simulink model "untitled1"  (R2022b)
settings: Solver=ode4  StartTime=0.0  StopTime=2  FixedStep=.01  RelTol=1e-3
settings Model: Creator=hp_desktop  LastModifiedBy=hp_desktop

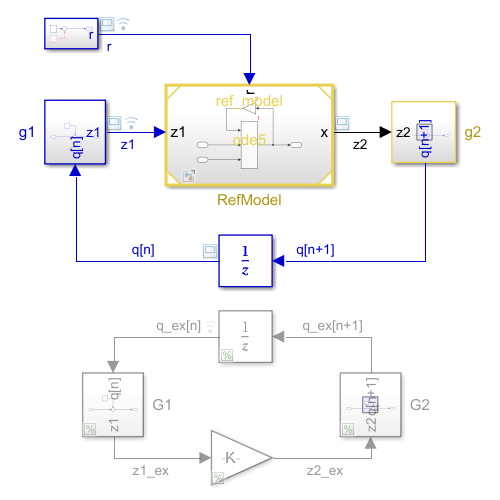
[thumbnail: Simulink's stored preview of the top-level diagram]
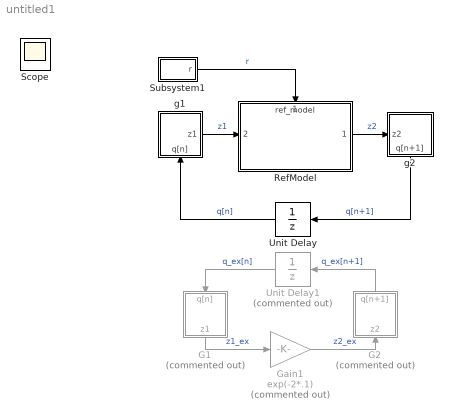
== system untitled1 ==
  G1 : Subsystem  Commented=on
      settings: PortSchema="{\"entries\":[{\"content\":{\"sides\":[{\"content\":{\"connectorIds\":[]},\"type\":\"ConnectorPlacement.EquallySpacedRectSide\",\"uuid\":\"86c8c839-e474-4a95-956c-b3cf1d577c6b\"},{\"content\":{\"connectorIds\":[],\"side\":\"RIGHT\"},\"type\":\"ConnectorPlacement.EquallySpacedRectSide\",\"uuid\":\"39481f83-4199-4de7-a4e8-5561103d4776\"},{\"content\":{\"connectorIds\":[\"Out1\"],\"side\":\"TOP\"},\"type\":\"ConnectorPlacement.EquallySpacedRectSide\",\"uuid\":\"ba4267bb-ac31-48a1-9c03-9fbc1cd5a7ee\"},{\"content\":{\"connectorIds\":[\"In1\"],\"side\":\"BOTTOM\"},\"type\":\"ConnectorPlacement.EquallySpacedRectSide\",\"uuid\":\"8bb6862b-83a9-47f6-8568-3761b0d351a6\"}]},\"type\":\"ConnectorPlacement.EquallySpacedConnector\",\"uuid\":\"7828d7b7-bf8b-4dbd-a99c-1d2acdedce65\"}],\"packageUris\":[\"http://schema.mathworks.com/mf0/Connector/R2020b\"],\"version\":\"1.0\"}"
  G2 : Subsystem  Commented=on
      settings: PortSchema="{\"entries\":[{\"content\":{\"sides\":[{\"content\":{\"connectorIds\":[]},\"type\":\"ConnectorPlacement.EquallySpacedRectSide\",\"uuid\":\"86c8c839-e474-4a95-956c-b3cf1d577c6b\"},{\"content\":{\"connectorIds\":[],\"side\":\"RIGHT\"},\"type\":\"ConnectorPlacement.EquallySpacedRectSide\",\"uuid\":\"39481f83-4199-4de7-a4e8-5561103d4776\"},{\"content\":{\"connectorIds\":[\"Out1\"],\"side\":\"TOP\"},\"type\":\"ConnectorPlacement.EquallySpacedRectSide\",\"uuid\":\"ba4267bb-ac31-48a1-9c03-9fbc1cd5a7ee\"},{\"content\":{\"connectorIds\":[\"In1\"],\"side\":\"BOTTOM\"},\"type\":\"ConnectorPlacement.EquallySpacedRectSide\",\"uuid\":\"8bb6862b-83a9-47f6-8568-3761b0d351a6\"}]},\"type\":\"ConnectorPlacement.EquallySpacedConnector\",\"uuid\":\"7828d7b7-bf8b-4dbd-a99c-1d2acdedce65\"}],\"packageUris\":[\"http://schema.mathworks.com/mf0/Connector/R2020b\"],\"version\":\"1.0\"}"
  Gain1 : Gain  Commented=on  Gain=exp(-2*.1)
  RefModel : ModelReference  ModelNameDialog=ref_model.slx  SimulationMode=Normal  ModelReferenceVersion=1.9
      settings: PortSchema="{\"entries\":[{\"content\":{\"sides\":[{\"content\":{\"connectorIds\":[\"In2\"]},\"type\":\"ConnectorPlacement.EquallySpacedRectSide\",\"uuid\":\"337a5834-4e8a-490b-adbc-054d163d2861\"},{\"content\":{\"connectorIds\":[\"Out1\"],\"side\":\"RIGHT\"},\"type\":\"ConnectorPlacement.EquallySpacedRectSide\",\"uuid\":\"5c62d075-0782-4b5e-908a-3bc3e009ebc7\"},{\"content\":{\"connectorIds\":[\"In1\"],\"side\":\"TOP\"},\"type\":\"ConnectorPlacement.EquallySpacedRectSide\",\"uuid\":\"4db60da9-bb5a-4f60-ab65-a5e9fb18bbef\"}]},\"type\":\"ConnectorPlacement.EquallySpacedConnector\",\"uuid\":\"e858c7ca-5f05-4367-a1a4-03373953631b\"}],\"packageUris\":[\"http://schema.mathworks.com/mf0/Connector/R2020b\"],\"version\":\"1.0\"}"
  Subsystem1 : Subsystem
  Unit Delay : UnitDelay  SampleTime=.1  HasFrameUpgradeWarning=on
  Unit Delay1 : UnitDelay  Commented=on  SampleTime=.1  HasFrameUpgradeWarning=on
  g1 : Subsystem
      settings: PortSchema="{\"entries\":[{\"content\":{\"sides\":[{\"content\":{\"connectorIds\":[]},\"type\":\"ConnectorPlacement.EquallySpacedRectSide\",\"uuid\":\"86c8c839-e474-4a95-956c-b3cf1d577c6b\"},{\"content\":{\"connectorIds\":[\"Out1\"],\"side\":\"RIGHT\"},\"type\":\"ConnectorPlacement.EquallySpacedRectSide\",\"uuid\":\"39481f83-4199-4de7-a4e8-5561103d4776\"},{\"content\":{\"connectorIds\":[],\"side\":\"TOP\"},\"type\":\"ConnectorPlacement.EquallySpacedRectSide\",\"uuid\":\"ba4267bb-ac31-48a1-9c03-9fbc1cd5a7ee\"},{\"content\":{\"connectorIds\":[\"In1\"],\"side\":\"BOTTOM\"},\"type\":\"ConnectorPlacement.EquallySpacedRectSide\",\"uuid\":\"8bb6862b-83a9-47f6-8568-3761b0d351a6\"}]},\"type\":\"ConnectorPlacement.EquallySpacedConnector\",\"uuid\":\"7828d7b7-bf8b-4dbd-a99c-1d2acdedce65\"}],\"packageUris\":[\"http://schema.mathworks.com/mf0/Connector/R2020b\"],\"version\":\"1.0\"}"
  g2 : Subsystem
      settings: PortSchema="{\"entries\":[{\"content\":{\"sides\":[{\"content\":{\"connectorIds\":[\"Out1\"]},\"type\":\"ConnectorPlacement.EquallySpacedRectSide\",\"uuid\":\"86c8c839-e474-4a95-956c-b3cf1d577c6b\"},{\"content\":{\"connectorIds\":[],\"side\":\"RIGHT\"},\"type\":\"ConnectorPlacement.EquallySpacedRectSide\",\"uuid\":\"39481f83-4199-4de7-a4e8-5561103d4776\"},{\"content\":{\"connectorIds\":[],\"side\":\"TOP\"},\"type\":\"ConnectorPlacement.EquallySpacedRectSide\",\"uuid\":\"ba4267bb-ac31-48a1-9c03-9fbc1cd5a7ee\"},{\"content\":{\"connectorIds\":[\"In1\"],\"side\":\"BOTTOM\"},\"type\":\"ConnectorPlacement.EquallySpacedRectSide\",\"uuid\":\"8bb6862b-83a9-47f6-8568-3761b0d351a6\"}]},\"type\":\"ConnectorPlacement.EquallySpacedConnector\",\"uuid\":\"7828d7b7-bf8b-4dbd-a99c-1d2acdedce65\"}],\"packageUris\":[\"http://schema.mathworks.com/mf0/Connector/R2020b\"],\"version\":\"1.0\"}"
  Scope : Scope
  wires:
  Unit Delay/1 -> g1/1(q[n])  "q[n]"
  g1/1(z1) -> RefModel/2  "z1"
  RefModel/1 -> g2/1(z2)  "z2"
  g2/1(q[n+1]) -> Unit Delay/1  "q[n+1]"
  Unit Delay1/1 -> G1/1(q[n])  "q_ex[n]"
  G1/1(z1) -> Gain1/1  "z1_ex"
  G2/1(q[n+1]) -> Unit Delay1/1  "q_ex[n+1]"
  Gain1/1 -> G2/1(z2)  "z2_ex"
  Subsystem1/1(r) -> RefModel/1  "r"

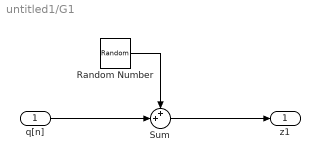
== system untitled1/G1 ==
  q[n] : Inport
  Random Number : RandomNumber  SampleTime=0.1
  Sum : Sum  Inputs=++|
  z1 : Outport
  wires:
  Random Number/1 -> Sum/1
  Sum/1 -> z1/1
  q[n]/1 -> Sum/2

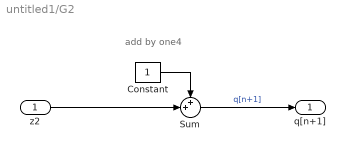
== system untitled1/G2 ==
  note: add by one4
  z2 : Inport
  Constant : Constant
  Sum : Sum  Inputs=++|
  q[n+1] : Outport
  wires:
  Sum/1 -> q[n+1]/1  "q[n+1]"
  z2/1 -> Sum/2
  Constant/1 -> Sum/1

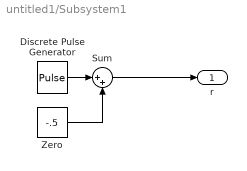
== system untitled1/Subsystem1 ==
  Discrete Pulse Generator : DiscretePulseGenerator  SampleTime=.1
  Sum : Sum  Inputs=|++
  Zero : Constant  Value=-.5  OutDataTypeStr=Inherit: Inherit via back propagation
  r : Outport
  wires:
  Sum/1 -> r/1
  Discrete Pulse Generator/1 -> Sum/1
  Zero/1 -> Sum/2

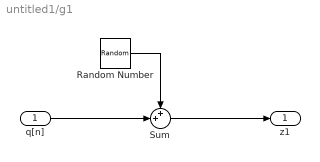
== system untitled1/g1 ==
  q[n] : Inport
  Random Number : RandomNumber  SampleTime=0.1
  Sum : Sum  Inputs=++|
  z1 : Outport
  wires:
  q[n]/1 -> Sum/2
  Sum/1 -> z1/1
  Random Number/1 -> Sum/1

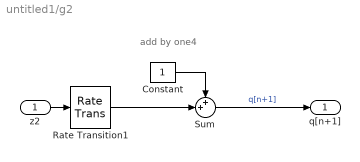
== system untitled1/g2 ==
  note: add by one4
  z2 : Inport
  Constant : Constant
  Rate Transition1 : RateTransition  OutPortSampleTime=.1
  Sum : Sum  Inputs=++|
  q[n+1] : Outport
  wires:
  Constant/1 -> Sum/1
  z2/1 -> Rate Transition1/1
  Sum/1 -> q[n+1]/1  "q[n+1]"
  Rate Transition1/1 -> Sum/2
